simulink library "WECSim_Lib_update"  (Simulink 8.6)
settings: Solver=ode45  StartTime=0.0  StopTime=10.0  RelTol=1e-3
undefined symbols (not defined in the file or in its folder): body, constraint, mooring, pto, simu, waves, X, Y, Z
libraries: nesl_utility x168, sm_lib x94, vrlib x1
(part 5 of 6)

== system WECSim_Lib_update/Body Elements/Rigid Body/Hydrodynamic Body/Structure/Motion Sensor ==
  note: Measures the position, velocity, and acceleration of the follower (F) frame relative to the base (B) frame.
      | Ouputs a bus of 3 signals, each signal is a vector length 6.
  Angle : MATLAB Function  TreatAsAtomicUnit=on
  Bus Creator : BusCreator  Inputs=3
  Mux : Mux
  Mux1 : Mux  Inputs=6
  Mux2 : Mux  Inputs=6
  PS-Simulink Converter{,1..15} (16 alike) : nesl_utility/PS-Simulink Converter  PhysicalDomain=network_engine_domain  SubClassName=ps_output  LeftPortType=input  RightPortType=output  PseudoPeriodic=off  Frequencies=[]  AffineConversion=off
  Transform  Sensor : sm_lib/Frames and Transforms/Transform Sensor  MeasurementFrame=World  SenseAngle=off  SenseAxis=off  SenseAngle1=off  SenseAngle2=off  SenseAngle3=off  SenseQ=on  SenseR=off  SenseOmegaX=on  SenseOmegaY=on  SenseOmegaZ=on  SenseOmega1=off  SenseOmega2=off  SenseOmega3=off  SenseQDot=off  SenseRDot=off  SenseAlphaX=on  SenseAlphaY=on  SenseAlphaZ=on  SenseAlpha1=off  SenseAlpha2=off  SenseAlpha3=off  SenseQDDot=off  SenseRDDot=off  SenseX=on  SenseY=on  SenseZ=on  SenseRad=off  SenseAzim=off  SenseDist=off  SenseInc=off  SenseXDot=on  SenseYDot=on  SenseZDot=on  SenseRadDot=off  SenseAzimDot=off  SenseDistDot=off  SenseIncDot=off  SenseXDDot=on  SenseYDDot=on  SenseZDDot=on  SenseRadDDot=off  SenseAzimDDot=off  SenseDistDDot=off  SenseIncDDot=off
  F : PMIOPort  Port=1  Side=Right
  B : PMIOPort  Port=2  Side=Left
  Response : Outport
  wires:
  Bus Creator/1 -> Response/1
  PS-Simulink Converter15/1 -> Mux2/3  "az"
  PS-Simulink Converter3/1 -> Mux1/6  "omegaz"
  PS-Simulink Converter11/1 -> Mux1/2  "vy"
  PS-Simulink Converter2/1 -> Mux1/5  "omegay"
  PS-Simulink Converter1/1 -> Mux1/4  "omegax"
  PS-Simulink Converter6/1 -> Mux2/6  "alphaz"
  PS-Simulink Converter5/1 -> Mux2/5  "alphay"
  PS-Simulink Converter9/1 -> Mux/3  "z"
  PS-Simulink Converter8/1 -> Mux/2  "y"
  PS-Simulink Converter7/1 -> Mux/1  "x"
  Angle/1(E) -> Mux/4
  Mux2/1 -> Bus Creator/3  "acc"
  Mux1/1 -> Bus Creator/2  "vel"
  Mux/1 -> Bus Creator/1  "disp"
  PS-Simulink Converter14/1 -> Mux2/2  "ay"
  PS-Simulink Converter13/1 -> Mux2/1  "ax"
  PS-Simulink Converter12/1 -> Mux1/3  "vz"
  PS-Simulink Converter10/1 -> Mux1/1  "vx"
  PS-Simulink Converter4/1 -> Mux2/4  "alphax"
  PS-Simulink Converter/1 -> Angle/1(Q)
  connections:
  PS-Simulink Converter3/LConn1 -- Transform  Sensor/RConn5
  PS-Simulink Converter2/LConn1 -- Transform  Sensor/RConn4
  PS-Simulink Converter1/LConn1 -- Transform  Sensor/RConn3
  PS-Simulink Converter6/LConn1 -- Transform  Sensor/RConn8
  PS-Simulink Converter5/LConn1 -- Transform  Sensor/RConn7
  PS-Simulink Converter4/LConn1 -- Transform  Sensor/RConn6
  PS-Simulink Converter7/LConn1 -- Transform  Sensor/RConn9
  PS-Simulink Converter8/LConn1 -- Transform  Sensor/RConn10
  PS-Simulink Converter9/LConn1 -- Transform  Sensor/RConn11
  PS-Simulink Converter10/LConn1 -- Transform  Sensor/RConn12
  PS-Simulink Converter11/LConn1 -- Transform  Sensor/RConn13
  PS-Simulink Converter12/LConn1 -- Transform  Sensor/RConn14
  PS-Simulink Converter13/LConn1 -- Transform  Sensor/RConn15
  PS-Simulink Converter14/LConn1 -- Transform  Sensor/RConn16
  PS-Simulink Converter15/LConn1 -- Transform  Sensor/RConn17
  Transform  Sensor/RConn2 -- PS-Simulink Converter/LConn1
  B/RConn1 -- Transform  Sensor/LConn1
  Transform  Sensor/RConn1 -- F/RConn1

== system WECSim_Lib_update/Body Elements/Rigid Body/Hydrodynamic Body/Wave Diffraction and Excitation Force Calculation/Linear Wave Excitation Force Variant Subsystem ==
  note: 1) Add Subsystem or Model blocks as valid variant choices.
      | 2) You cannot connect blocks at this level. At simulation, connectivity is automatically
      | determined, based on the active variant and port name matching.
  In1 : Inport
  Irregular Wave  Excitation Force : Subsystem  VariantControl=sv_irregularWaves
  No Wave Excitation Force : Subsystem  VariantControl=sv_noWave
  Regular Wave  Excitation Force : Subsystem  VariantControl=sv_regularWaves
  User Defined Wave  Excitation Force : Subsystem  VariantControl=sv_udfWaves
  Out1 : Outport

== system WECSim_Lib_update/Body Elements/Rigid Body/Hydrodynamic Body/Wave Diffraction and Excitation Force Calculation/No Ramp Function ==
  Action Port : ActionPort
  Constant : Constant
  R : Outport  InitialOutput=1
  wires:
  Constant/1 -> R/1

== system WECSim_Lib_update/Body Elements/Rigid Body/Hydrodynamic Body/Wave Diffraction and Excitation Force Calculation/Nonlinear FK Force Variant Subsystem ==
  note: 1) Add Subsystem or Model blocks as valid variant choices.
      | 2) You cannot connect blocks at this level. At simulation, connectivity is automatically
      | determined, based on the active variant and port name matching.
  In1 : Inport
  In2 : Inport  Port=2
  In3 : Inport  Port=3
  No Nonlinear FroudeKrylov Force : Subsystem  VariantControl=sv_linearHydro
  With Nonlinear FroudeKrylov Force : Subsystem  TreatAsAtomicUnit=on  SystemSampleTime=simu.dtNL  VariantControl=sv_nonlinearHydro
  Out1 : Outport

== system WECSim_Lib_update/Body Elements/Rigid Body/Hydrodynamic Body/Wave Diffraction and Excitation Force Calculation/Ramp Function ==
  Time : Inport
  Action Port : ActionPort
  Add : Sum
  Add1 : Sum
  Constant : Constant  Value=1/2
  Constant1 : Constant
  Constant2 : Constant  Value=3*pi/2
  Constant3 : Constant  Value=pi
  Divide : Product  Inputs=*/
  Product : Product
  Product1 : Product
  Ramp Time : Constant  Value=simu.rampTime
  Sine Wave Function : Sin  TimeSource=Use external signal  SampleTime=0
  R : Outport
  wires:
  Add/1 -> Product/1
  Sine Wave Function/1 -> Add/2
  Constant1/1 -> Add/1
  Constant/1 -> Product/2
  Product/1 -> R/1
  Time/1 -> Product1/1  "t"
  Ramp Time/1 -> Divide/2  "t_ramp"
  Constant2/1 -> Add1/2  "phase"
  Add1/1 -> Sine Wave Function/1
  Product1/1 -> Add1/1
  Constant3/1 -> Divide/1
  Divide/1 -> Product1/2  "frequency"

== system WECSim_Lib_update/Body Elements/Rigid Body/Hydrodynamic Body/Wave Radiation Forces Calculation/SS CI and Constant-Damping-CoeVariant Subsystem ==
  note: 1) Add Subsystem or Model blocks as valid variant choices.
      | 2) You cannot connect blocks at this level. At simulation, connectivity is automatically
      | determined, based on the active variant and port name matching.
  In1 : Inport
  In2 : Inport  Port=2
  Constant Coefficients : Subsystem  VariantControl=sv_constantCoeff
  Convolution Integral Calculation : Subsystem  VariantControl=sv_convolution
  "State-Space Calculation " : Subsystem  VariantControl=sv_stateSpace
  Out1 : Outport

== system WECSim_Lib_update/Body Elements/Rigid Body/Non-Hydro Body/Structure/Motion Sensor ==
  note: Measures the position, velocity, and acceleration of the follower (F) frame relative to the base (B) frame.
      | Ouputs a bus of 3 signals, each signal is a vector length 6.
  Angle : MATLAB Function  TreatAsAtomicUnit=on
  Bus Creator : BusCreator  Inputs=3
  Mux : Mux
  Mux1 : Mux  Inputs=6
  Mux2 : Mux  Inputs=6
  PS-Simulink Converter{,1..15} (16 alike) : nesl_utility/PS-Simulink Converter  PhysicalDomain=network_engine_domain  SubClassName=ps_output  LeftPortType=input  RightPortType=output  PseudoPeriodic=off  Frequencies=[]  AffineConversion=off
  Transform  Sensor : sm_lib/Frames and Transforms/Transform Sensor  MeasurementFrame=World  SenseAngle=off  SenseAxis=off  SenseAngle1=off  SenseAngle2=off  SenseAngle3=off  SenseQ=on  SenseR=off  SenseOmegaX=on  SenseOmegaY=on  SenseOmegaZ=on  SenseOmega1=off  SenseOmega2=off  SenseOmega3=off  SenseQDot=off  SenseRDot=off  SenseAlphaX=on  SenseAlphaY=on  SenseAlphaZ=on  SenseAlpha1=off  SenseAlpha2=off  SenseAlpha3=off  SenseQDDot=off  SenseRDDot=off  SenseX=on  SenseY=on  SenseZ=on  SenseRad=off  SenseAzim=off  SenseDist=off  SenseInc=off  SenseXDot=on  SenseYDot=on  SenseZDot=on  SenseRadDot=off  SenseAzimDot=off  SenseDistDot=off  SenseIncDot=off  SenseXDDot=on  SenseYDDot=on  SenseZDDot=on  SenseRadDDot=off  SenseAzimDDot=off  SenseDistDDot=off  SenseIncDDot=off
  F : PMIOPort  Port=1  Side=Right
  B : PMIOPort  Port=2  Side=Left
  Response : Outport
  wires:
  Bus Creator/1 -> Response/1
  PS-Simulink Converter15/1 -> Mux2/3  "az"
  PS-Simulink Converter3/1 -> Mux1/6  "omegaz"
  PS-Simulink Converter11/1 -> Mux1/2  "vy"
  PS-Simulink Converter2/1 -> Mux1/5  "omegay"
  PS-Simulink Converter1/1 -> Mux1/4  "omegax"
  PS-Simulink Converter6/1 -> Mux2/6  "alphaz"
  PS-Simulink Converter5/1 -> Mux2/5  "alphay"
  PS-Simulink Converter9/1 -> Mux/3  "z"
  PS-Simulink Converter8/1 -> Mux/2  "y"
  PS-Simulink Converter7/1 -> Mux/1  "x"
  Angle/1(E) -> Mux/4
  Mux2/1 -> Bus Creator/3  "acc"
  Mux1/1 -> Bus Creator/2  "vel"
  Mux/1 -> Bus Creator/1  "disp"
  PS-Simulink Converter14/1 -> Mux2/2  "ay"
  PS-Simulink Converter13/1 -> Mux2/1  "ax"
  PS-Simulink Converter12/1 -> Mux1/3  "vz"
  PS-Simulink Converter10/1 -> Mux1/1  "vx"
  PS-Simulink Converter4/1 -> Mux2/4  "alphax"
  PS-Simulink Converter/1 -> Angle/1(Q)
  connections:
  PS-Simulink Converter3/LConn1 -- Transform  Sensor/RConn5
  PS-Simulink Converter2/LConn1 -- Transform  Sensor/RConn4
  PS-Simulink Converter1/LConn1 -- Transform  Sensor/RConn3
  PS-Simulink Converter6/LConn1 -- Transform  Sensor/RConn8
  PS-Simulink Converter5/LConn1 -- Transform  Sensor/RConn7
  PS-Simulink Converter4/LConn1 -- Transform  Sensor/RConn6
  PS-Simulink Converter7/LConn1 -- Transform  Sensor/RConn9
  PS-Simulink Converter8/LConn1 -- Transform  Sensor/RConn10
  PS-Simulink Converter9/LConn1 -- Transform  Sensor/RConn11
  PS-Simulink Converter10/LConn1 -- Transform  Sensor/RConn12
  PS-Simulink Converter11/LConn1 -- Transform  Sensor/RConn13
  PS-Simulink Converter12/LConn1 -- Transform  Sensor/RConn14
  PS-Simulink Converter13/LConn1 -- Transform  Sensor/RConn15
  PS-Simulink Converter14/LConn1 -- Transform  Sensor/RConn16
  PS-Simulink Converter15/LConn1 -- Transform  Sensor/RConn17
  Transform  Sensor/RConn2 -- PS-Simulink Converter/LConn1
  B/RConn1 -- Transform  Sensor/LConn1
  Transform  Sensor/RConn1 -- F/RConn1

== system WECSim_Lib_update/Moorings/MoorDyn/MoorDyn/MoorDyn/Triggered Subsystem ==
  X : Inport
  XD : Inport  Port=2
  Time : Inport  Port=3
  CoupTime : Inport  Port=4
  Trigger : TriggerPort  TriggerType=either
  MATLAB Function : MATLAB Function  TreatAsAtomicUnit=on
  FLines : Outport  PortDimensions=6
  wires:
  CoupTime/1 -> MATLAB Function/4(CoupTime)
  Time/1 -> MATLAB Function/3(Time)
  XD/1 -> MATLAB Function/2(XD)
  MATLAB Function/1(FLines) -> FLines/1
  X/1 -> MATLAB Function/1(X)

== system WECSim_Lib_update/Body Elements/Rigid Body/Hydrodynamic Body/B2B Subsystem/B2B/CrossCoupling ==
  note: CrossCoupling block is updated by its mask initialization, which is only called on when a simulation is run. 'From' blocks are automatically created and connected based on the number of bodies in the simulation.
  Mux1 : Mux  Inputs=2
  Mux2 : Mux  Inputs=2
  vel : Outport
  acc : Outport  Port=2
  wires:
  [vel1] -> Mux1/1
  Mux1/1 -> vel/1
  [vel2] -> Mux1/2
  [acc1] -> Mux2/1
  Mux2/1 -> acc/1
  [acc2] -> Mux2/2

== system WECSim_Lib_update/Body Elements/Rigid Body/Hydrodynamic Body/Hydrostatic Restoring Force Calculation/Linear and Nonlinear Restoring Force Variant Subsystem/Linear Hydrostatic Restoring Force  ==
  In1 : Inport
  Add1 : Sum  Inputs=+-
  Add2 : Sum  Inputs=+++
  Add3 : Sum  Inputs=+-
  Assignment (Add Net Bouyancy Force  to Z-Direction) : Assignment  IndexOptions=Index vector (dialog)  Indices=3  OutputSizes=1
  Assignment (Add Net Bouyancy Force  to Z-Direction)1 : Assignment  IndexOptions=Index vector (dialog)  Indices=3  OutputSizes=1
  Assignment (Add Net Bouyancy Force  to Z-Direction)2 : Assignment  IndexOptions=Index vector (dialog)  Indices=4:6  OutputSizes=1
  Body Mass : Constant  Value=body.hydroForce.storage.mass
  Center of Buoyancy : Constant  Value=body.cb
  Center of Gravity : Constant  Value=body.cg
  Constant1 : Constant  Value=[0 0 0 0 0 0]
  Constant2 : Constant  Value=[0 0 0]
  Cross Product : vrlib/Utilities/Cross Product
  Gravity : Constant  Value=simu.g
  Linear Restioring Coefficient Matrix : Constant  Value=body.hydroForce.linearHydroRestCoef
  Product : Product
  Product1 : Product  Inputs=3
  Product2 : Product  Multiplication=Matrix(*)
  Volume : Constant  Value=body.dispVol
  Water Density : Constant  Value=simu.rho
  Out1 : Outport
  wires:
  In1/1 -> Product2/2  "x"
  Body Mass/1 -> Product/2  "m"
  Assignment (Add Net Bouyancy Force  to Z-Direction)/1 -> Add2/1  "Net Buoyancy Force"
  Add2/1 -> Out1/1  "F_Restoring"
  Volume/1 -> Product1/3  "Vol"
  Gravity/1 -> Product1/2, Product/1  "g"
  Water Density/1 -> Product1/1  "rho"
  Product/1 -> Add1/1  "F_Gravity"
  Product1/1 -> Add1/2, Assignment (Add Net Bouyancy Force  to Z-Direction)1/2  "F_Buoyancy"
  Add1/1 -> Assignment (Add Net Bouyancy Force  to Z-Direction)/2
  Product2/1 -> Add2/2  "Linear Restoring Force"
  Linear Restioring Coefficient Matrix/1 -> Product2/1  "K"
  Center of Buoyancy/1 -> Add3/1  "x"
  Center of Gravity/1 -> Add3/2  "cg"
  Add3/1 -> Cross Product/2
  Constant2/1 -> Assignment (Add Net Bouyancy Force  to Z-Direction)1/1
  Assignment (Add Net Bouyancy Force  to Z-Direction)1/1 -> Cross Product/1
  Cross Product/1 -> Assignment (Add Net Bouyancy Force  to Z-Direction)2/2
  Constant1/1 -> Assignment (Add Net Bouyancy Force  to Z-Direction)2/1, Assignment (Add Net Bouyancy Force  to Z-Direction)/1
  Assignment (Add Net Bouyancy Force  to Z-Direction)2/1 -> Add2/3

== system WECSim_Lib_update/Body Elements/Rigid Body/Hydrodynamic Body/Hydrostatic Restoring Force Calculation/Linear and Nonlinear Restoring Force Variant Subsystem/Nonlinear Hydrostatic Restoring Force ==
  In1 : Inport
  In2 : Inport  Port=2
  Body Mass2 : Constant  Value=body.hydroForce.storage.mass
  Center of Gravity : Constant  Value=body.cg
  Gravity2 : Constant  Value=simu.g
  Rate Transition : RateTransition
  Rate Transition1 : RateTransition
  Restoring Forces : MATLAB Function  TreatAsAtomicUnit=on  SystemSampleTime=simu.dtNL
  STL areas : Constant  Value=body.bodyGeometry.area
  STL centers : Constant  Value=body.bodyGeometry.center
  STL normal vectors : Constant  Value=body.bodyGeometry.norm
  To Workspace1 : ToWorkspace  VariableName=body1_hspressure_out  SaveFormat=Structure With Time  SampleTime=-1
      settings: Decimation=round(simu.dtOut/simu.dt,0)
  Water Density1 : Constant  Value=simu.rho
  Out1 : Outport
  wires:
  In1/1 -> Restoring Forces/1(x)
  Center of Gravity/1 -> Restoring Forces/8(cg)
  Gravity2/1 -> Restoring Forces/7(g)  "g"
  Water Density1/1 -> Restoring Forces/6(rho)
  STL normal vectors/1 -> Restoring Forces/4(tnorm)
  STL centers/1 -> Restoring Forces/3(center)
  In2/1 -> Restoring Forces/2(elv)
  STL areas/1 -> Restoring Forces/5(area)
  Body Mass2/1 -> Restoring Forces/9(mass)
  Restoring Forces/2(p) -> Rate Transition1/1
  Rate Transition1/1 -> To Workspace1/1
  Restoring Forces/1(f) -> Rate Transition/1
  Rate Transition/1 -> Out1/1

== system WECSim_Lib_update/Body Elements/Rigid Body/Hydrodynamic Body/Morrison Element and ViscousDampingForceCalculation/Morrison Element Variant Subsystem/Morrison Element Off ==
  Constant : Constant  Value=[0 0 0 0 0 0]
  morison_force : Outport
  wires:
  Constant/1 -> morison_force/1

== system WECSim_Lib_update/Body Elements/Rigid Body/Hydrodynamic Body/Morrison Element and ViscousDampingForceCalculation/Morrison Element Variant Subsystem/Morrison Element On ==
  note: 1) Add Subsystem or Model blocks as valid variant choices.
      | 2) You cannot connect blocks at this level. At simulation, connectivity is automatically
      | determined, based on the active variant and port name matching.
  displacement : Inport
  velocity : Inport  Port=2
  acceleration : Inport  Port=3
  time : Inport  Port=4
  Irregular Wave  Morison Force : Subsystem  TreatAsAtomicUnit=on  SystemSampleTime=simu.dtME  VariantControl=sv_irregularWaves
  No Wave Morison Force : Subsystem  VariantControl=sv_noWave
  Regular Wave  Morison Force : Subsystem  TreatAsAtomicUnit=on  SystemSampleTime=simu.dtME  VariantControl=sv_regularWaves
  morison_force : Outport

== system WECSim_Lib_update/Body Elements/Rigid Body/Hydrodynamic Body/Nonlinear Wave Elevation/Linear or Instantaneous Free Surface/Instantaneous Water Free Surface   ==
  In1 : Inport
  In2 : Inport  Port=2
  Center of Gravity : Constant  Value=body.cg
  Frequency Spacing : Constant  Value=waves.dw
  Instantaneous FS : MATLAB Function  TreatAsAtomicUnit=on
  Ramp Time : Constant  Value=simu.rampTime
  STL Centers : Constant  Value=body.bodyGeometry.center
  Wave Amplitude : Constant  Value=waves.A
  Wave Direction : Constant  Value=waves.waveDir
  Wave Frequency : Constant  Value=waves.w
  Wave Number : Constant  Value=waves.k
  Wave Random Phase : Constant  Value=waves.phase
  Wave Type Number : Constant  Value=waves.typeNum
  Out1 : Outport
  wires:
  Instantaneous FS/1(f) -> Out1/1
  STL Centers/1 -> Instantaneous FS/2(center)
  Center of Gravity/1 -> Instantaneous FS/3(cg)
  Wave Number/1 -> Instantaneous FS/7(k)
  Wave Frequency/1 -> Instantaneous FS/5(w)
  Wave Type Number/1 -> Instantaneous FS/8(typeNum)
  Ramp Time/1 -> Instantaneous FS/10(rampT)
  Wave Random Phase/1 -> Instantaneous FS/11(phaseRand)
  Frequency Spacing/1 -> Instantaneous FS/6(dw)
  In2/1 -> Instantaneous FS/9(t)
  In1/1 -> Instantaneous FS/1(x)
  Wave Direction/1 -> Instantaneous FS/12(waveDir)
  Wave Amplitude/1 -> Instantaneous FS/4(AH)

== system WECSim_Lib_update/Body Elements/Rigid Body/Hydrodynamic Body/Nonlinear Wave Elevation/Linear or Instantaneous Free Surface/Mean Water Free Surface  ==
  zero : Constant  Value=0
  Out1 : Outport
  wires:
  zero/1 -> Out1/1

== system WECSim_Lib_update/Body Elements/Rigid Body/Hydrodynamic Body/Wave Diffraction and Excitation Force Calculation/Linear Wave Excitation Force Variant Subsystem/Irregular Wave  Excitation Force ==
  note: Calculates the wave force, F_wave, for the case of Irregular Waves.
      |
      | F_wave = sum( F_wave(i))
      |
      | where i = each frequency bin.
  In1 : Inport
  Frequency Spacing Delta Omega : Constant  Value=waves.dw  VectorParams1D=off
  Imaginary Part of Wave Excitation : Constant  Value=body.hydroForce.fExt.im  VectorParams1D=off
  MATLAB Function : MATLAB Function  TreatAsAtomicUnit=on
  Random Phase : Constant  Value=waves.phase  VectorParams1D=off
  Real Part of Wave Excitation : Constant  Value=body.hydroForce.fExt.re  VectorParams1D=off
  Wave Frequency : Constant  Value=waves.w  VectorParams1D=off
  Wave Spectrum : Constant  Value=waves.A  VectorParams1D=off
  Out1 : Outport
  wires:
  Random Phase/1 -> MATLAB Function/5(phaseRand)
  MATLAB Function/1(Fext) -> Out1/1
  Wave Frequency/1 -> MATLAB Function/2(w)
  Imaginary Part of Wave Excitation/1 -> MATLAB Function/4(fExtIM)
  Real Part of Wave Excitation/1 -> MATLAB Function/3(fExtRE)
  Wave Spectrum/1 -> MATLAB Function/1(A)
  In1/1 -> MATLAB Function/7(time)
  Frequency Spacing Delta Omega/1 -> MATLAB Function/6(dw)

== system WECSim_Lib_update/Body Elements/Rigid Body/Hydrodynamic Body/Wave Diffraction and Excitation Force Calculation/Linear Wave Excitation Force Variant Subsystem/No Wave Excitation Force ==
  Constant : Constant  Value=[0 0 0 0 0 0]
  Out1 : Outport
  wires:
  Constant/1 -> Out1/1

== system WECSim_Lib_update/Body Elements/Rigid Body/Hydrodynamic Body/Wave Diffraction and Excitation Force Calculation/Linear Wave Excitation Force Variant Subsystem/Regular Wave  Excitation Force ==
  note: Calculates the wave force, F_wave, for the case of Regular Waves.
      |
      | F_wave =   A * cos(w * t) * Re{Fext}
      |                -  A * sin(w * t) * Im{Fext}
  In1 : Inport
  Add : Sum
  Add1 : Sum  Inputs=+-
  Constant : Constant  Value=pi/2
  Excitation Imaginary Part : Constant  Value=body.hydroForce.fExt.im(1,:)  VectorParams1D=off
  Excitation Real Part : Constant  Value=body.hydroForce.fExt.re(1,:)  VectorParams1D=off
  Product : Product
  Product1 : Product  Inputs=3
  Product2 : Product  Inputs=3
  Sine Wave Function : Sin  TimeSource=Use external signal  SampleTime=0
  Sine Wave Function1 : Sin  TimeSource=Use external signal  SampleTime=0
  Wave Amplitude : Constant  Value=waves.A(1,:)
  Wave Frequency : Constant  Value=waves.w(1,:)
  Out1 : Outport
  wires:
  In1/1 -> Product/1  "t"
  Wave Frequency/1 -> Product/2  "w"
  Product/1 -> Sine Wave Function/1, Add/1
  Sine Wave Function1/1 -> Product1/3  "cos(w*t)"
  Sine Wave Function/1 -> Product2/2  "sin(wt)"
  Excitation Imaginary Part/1 -> Product2/3  "Im{Fext}"
  Excitation Real Part/1 -> Product1/2  "Re{Fext}"
  Product1/1 -> Add1/1
  Product2/1 -> Add1/2
  Add1/1 -> Out1/1
  Wave Amplitude/1 -> Product2/1, Product1/1  "A"
  Add/1 -> Sine Wave Function1/1
  Constant/1 -> Add/2

== system WECSim_Lib_update/Body Elements/Rigid Body/Hydrodynamic Body/Wave Diffraction and Excitation Force Calculation/Linear Wave Excitation Force Variant Subsystem/User Defined Wave  Excitation Force ==
  note: Calculates the wave force, F_wave, for the case of User Defined Waves.
      |
      | F_wave = convolution calculation [1x6]
  InputWaveForceTimeHistory : FromWorkspace  VariableName=[waves.waveAmpTime(:,1),body.hydroForce.userDefinedFe]  SampleTime=0
  Out1 : Outport
  wires:
  InputWaveForceTimeHistory/1 -> Out1/1

== system WECSim_Lib_update/Body Elements/Rigid Body/Hydrodynamic Body/Wave Diffraction and Excitation Force Calculation/Nonlinear FK Force Variant Subsystem/No Nonlinear FroudeKrylov Force ==
  Constant : Constant  Value=[0 0 0 0 0 0]
  Out1 : Outport
  wires:
  Constant/1 -> Out1/1

== system WECSim_Lib_update/Body Elements/Rigid Body/Hydrodynamic Body/Wave Diffraction and Excitation Force Calculation/Nonlinear FK Force Variant Subsystem/With Nonlinear FroudeKrylov Force ==
  In1 : Inport
  In2 : Inport  Port=2
  In3 : Inport  Port=3
  Add : Sum  Inputs=+-
  Center of Gravity : Constant  Value=body.hydroData.properties.cg
  Center of Gravity1 : Constant  Value=body.hydroData.properties.cg
  Constant : Constant  Value=[0 0 0]
  Deep Water Flag : Constant  Value=waves.deepWaterWave
  Diffraction and Excitation Forces : MATLAB Function  TreatAsAtomicUnit=on
  Frequency Spacing : Constant  Value=waves.dw
  Gravity : Constant  Value=simu.g
  Mux : Mux  Inputs=2
  STL Areas : Constant  Value=body.bodyGeometry.area
  STL Centers : Constant  Value=body.bodyGeometry.center
  STL Normal Vectors : Constant  Value=body.bodyGeometry.norm
  To Workspace : ToWorkspace  VariableName=body1_wavenonlinearpressure_out  SaveFormat=Structure With Time  SampleTime=-1
      settings: Decimation=round(simu.dtOut/simu.dt,0)
  To Workspace1 : ToWorkspace  VariableName=body1_wavelinearpressure_out  SaveFormat=Structure With Time  SampleTime=-1
      settings: Decimation=round(simu.dtOut/simu.dt,0)
  Water Density : Constant  Value=simu.rho
  Water Depth : Constant  Value=waves.waterDepth
  Wave Amplitude : Constant  Value=waves.A
  Wave Frequency : Constant  Value=waves.w
  Wave Number : Constant  Value=waves.k
  Wave Random Phase : Constant  Value=waves.phase
  Wave Type Number : Constant  Value=waves.typeNum
  Out1 : Outport
  wires:
  Center of Gravity1/1 -> Diffraction and Excitation Forces/8(cg)
  Diffraction and Excitation Forces/1(f) -> Out1/1
  Gravity/1 -> Diffraction and Excitation Forces/7(g)
  Water Density/1 -> Diffraction and Excitation Forces/6(rho)
  STL Normal Vectors/1 -> Diffraction and Excitation Forces/4(tnorm)
  STL Centers/1 -> Diffraction and Excitation Forces/3(center)
  In3/1 -> Diffraction and Excitation Forces/2(elv)
  In1/1 -> Diffraction and Excitation Forces/16(t)
  Wave Amplitude/1 -> Diffraction and Excitation Forces/9(AH)
  Wave Frequency/1 -> Diffraction and Excitation Forces/10(w)
  Frequency Spacing/1 -> Diffraction and Excitation Forces/11(dw)
  Wave Type Number/1 -> Diffraction and Excitation Forces/15(typeNum)
  Wave Number/1 -> Diffraction and Excitation Forces/14(k)
  Water Depth/1 -> Diffraction and Excitation Forces/12(wDepth)
  Wave Random Phase/1 -> Diffraction and Excitation Forces/17(phaseRand)
  Deep Water Flag/1 -> Diffraction and Excitation Forces/13(deepWaterWave)
  Add/1 -> Diffraction and Excitation Forces/1(x)  "x_cg"
  Mux/1 -> Add/2
  Center of Gravity/1 -> Mux/1  "cg"
  Constant/1 -> Mux/2
  In2/1 -> Add/1
  Diffraction and Excitation Forces/3(wpMeanFS) -> To Workspace1/1
  Diffraction and Excitation Forces/2(wp) -> To Workspace/1
  STL Areas/1 -> Diffraction and Excitation Forces/5(area)

== system WECSim_Lib_update/Body Elements/Rigid Body/Hydrodynamic Body/Wave Radiation Forces Calculation/SS CI and Constant-Damping-CoeVariant Subsystem/Constant Coefficients ==
  In1 : Inport
  Product : Product  Multiplication=Matrix(*)
  Radiation Damping Matrix : Constant  Value=body.hydroForce.fDamping
  Out1 : Outport
  wires:
  Radiation Damping Matrix/1 -> Product/1
  Product/1 -> Out1/1  "F_Single Frequency"
  In1/1 -> Product/2

== system WECSim_Lib_update/Body Elements/Rigid Body/Hydrodynamic Body/Wave Radiation Forces Calculation/SS CI and Constant-Damping-CoeVariant Subsystem/Convolution Integral Calculation ==
  In1 : Inport
  MATLAB Function : MATLAB Function  TreatAsAtomicUnit=on  SystemSampleTime=simu.CTTime(2) - simu.CTTime(1)  mask{IRKB=body.hydroForce.irkb, lenJ=length(body.lenJ), CTTime=simu.CTTime}
  Rate Transition : RateTransition
  Reshape : Reshape
  Out1 : Outport
  wires:
  In1/1 -> MATLAB Function/1(v)
  Reshape/1 -> Out1/1
  MATLAB Function/1(F_FM) -> Rate Transition/1
  Rate Transition/1 -> Reshape/1

== system WECSim_Lib_update/Body Elements/Rigid Body/Hydrodynamic Body/Wave Radiation Forces Calculation/SS CI and Constant-Damping-CoeVariant Subsystem/State-Space Calculation  ==
  In1 : Inport
  State-Space : StateSpace  A=body.hydroForce.ssRadf.A  B=body.hydroForce.ssRadf.B  C=body.hydroForce.ssRadf.C  D=body.hydroForce.ssRadf.D  X0=0
  Out1 : Outport
  wires:
  In1/1 -> State-Space/1  "x"
  State-Space/1 -> Out1/1

== system WECSim_Lib_update/Body Elements/Rigid Body/Hydrodynamic Body/Morrison Element and ViscousDampingForceCalculation/Morrison Element Variant Subsystem/Morrison Element On/Irregular Wave  Morison Force ==
  displacement : Inport
  velocity : Inport  Port=2
  acceleration : Inport  Port=3
  time : Inport  Port=4
  Area : Constant  Value=body.morrisonElement.characteristicArea  VectorParams1D=off
  Ca : Constant  Value=body.morrisonElement.ca  VectorParams1D=off
  Cd : Constant  Value=body.morrisonElement.cd  VectorParams1D=off
  Density : Constant  Value=simu.rho
  Gravity : Constant  Value=simu.g
  "MorrisonElement(s) " : MATLAB Function  TreatAsAtomicUnit=on
  Ramp Function Time : Constant  Value=simu.rampTime
  RandomPhaseAngle : Constant  Value=waves.phase  VectorParams1D=off
  Volume : Constant  Value=body.morrisonElement.VME  VectorParams1D=off
  WaterDepth : Constant  Value=waves.waterDepth
  WaveAmp : Constant  Value=waves.A
  WaveFreq : Constant  Value=waves.w
  WaveHeading : Constant  Value=waves.waveDir
  WaveNumber : Constant  Value=waves.k
  dw : Constant  Value=waves.dw  VectorParams1D=off
  "r_{g}" : Constant  Value=body.morrisonElement.rgME  VectorParams1D=off
  morison_force : Outport
  wires:
  Volume/1 -> "MorrisonElement(s) "/7(Vol)
  acceleration/1 -> "MorrisonElement(s) "/3(Accel)
  displacement/1 -> "MorrisonElement(s) "/4(Disp)
  Area/1 -> "MorrisonElement(s) "/5(Area)
  "r_{g}"/1 -> "MorrisonElement(s) "/1(r)
  velocity/1 -> "MorrisonElement(s) "/2(Vel)
  WaterDepth/1 -> "MorrisonElement(s) "/12(waterDepth)
  Gravity/1 -> "MorrisonElement(s) "/17(g)
  WaveNumber/1 -> "MorrisonElement(s) "/13(k)
  WaveHeading/1 -> "MorrisonElement(s) "/11(waveDir)
  time/1 -> "MorrisonElement(s) "/9(Time)
  Density/1 -> "MorrisonElement(s) "/10(rho)
  RandomPhaseAngle/1 -> "MorrisonElement(s) "/18(randPhase)
  WaveFreq/1 -> "MorrisonElement(s) "/14(w)
  Ca/1 -> "MorrisonElement(s) "/8(Ca)
  dw/1 -> "MorrisonElement(s) "/19(dw)
  WaveAmp/1 -> "MorrisonElement(s) "/15(A)
  Cd/1 -> "MorrisonElement(s) "/6(Cd)
  Ramp Function Time/1 -> "MorrisonElement(s) "/16(rampTime)
  "MorrisonElement(s) "/1(f) -> morison_force/1

== system WECSim_Lib_update/Body Elements/Rigid Body/Hydrodynamic Body/Morrison Element and ViscousDampingForceCalculation/Morrison Element Variant Subsystem/Morrison Element On/No Wave Morison Force ==
  displacement : Inport
  velocity : Inport  Port=2
  acceleration : Inport  Port=3
  time : Inport  Port=4
  Area : Constant  Value=body.morrisonElement.characteristicArea  VectorParams1D=off
  Ca : Constant  Value=body.morrisonElement.ca  VectorParams1D=off
  Cd : Constant  Value=body.morrisonElement.cd  VectorParams1D=off
  Density : Constant  Value=simu.rho
  "MorrisonElement(s) " : MATLAB Function  TreatAsAtomicUnit=on
  Terminator : Terminator
  Volume : Constant  Value=body.morrisonElement.VME  VectorParams1D=off
  "r_{g}" : Constant  Value=body.morrisonElement.rgME  VectorParams1D=off
  morison_force : Outport
  wires:
  "MorrisonElement(s) "/1(f) -> morison_force/1
  acceleration/1 -> "MorrisonElement(s) "/3(Accel)
  Density/1 -> "MorrisonElement(s) "/9(rho)
  Volume/1 -> "MorrisonElement(s) "/7(Vol)
  "r_{g}"/1 -> "MorrisonElement(s) "/1(r)
  Ca/1 -> "MorrisonElement(s) "/8(Ca)
  Area/1 -> "MorrisonElement(s) "/5(Area)
  displacement/1 -> "MorrisonElement(s) "/4(Disp)
  Cd/1 -> "MorrisonElement(s) "/6(Cd)
  velocity/1 -> "MorrisonElement(s) "/2(Vel)
  time/1 -> Terminator/1

== system WECSim_Lib_update/Body Elements/Rigid Body/Hydrodynamic Body/Morrison Element and ViscousDampingForceCalculation/Morrison Element Variant Subsystem/Morrison Element On/Regular Wave  Morison Force ==
  displacement : Inport
  velocity : Inport  Port=2
  acceleration : Inport  Port=3
  time : Inport  Port=4
  Area : Constant  Value=body.morrisonElement.characteristicArea  VectorParams1D=off
  Ca : Constant  Value=body.morrisonElement.ca  VectorParams1D=off
  Cd : Constant  Value=body.morrisonElement.cd  VectorParams1D=off
  Density : Constant  Value=simu.rho
  Gravity : Constant  Value=simu.g
  "MorrisonElement(s) " : MATLAB Function  TreatAsAtomicUnit=on
  Ramp Function Time : Constant  Value=simu.rampTime
  Volume : Constant  Value=body.morrisonElement.VME  VectorParams1D=off
  WaterDepth : Constant  Value=waves.waterDepth
  WaveAmp : Constant  Value=waves.A
  WaveFreq : Constant  Value=waves.w
  WaveHeading : Constant  Value=waves.waveDir
  WaveNumber : Constant  Value=waves.k
  "r_{g}" : Constant  Value=body.morrisonElement.rgME  VectorParams1D=off
  morison_force : Outport
  wires:
  "MorrisonElement(s) "/1(f) -> morison_force/1
  Volume/1 -> "MorrisonElement(s) "/7(Vol)
  Ca/1 -> "MorrisonElement(s) "/8(Ca)
  Gravity/1 -> "MorrisonElement(s) "/17(g)
  Cd/1 -> "MorrisonElement(s) "/6(Cd)
  displacement/1 -> "MorrisonElement(s) "/4(Disp)
  WaveAmp/1 -> "MorrisonElement(s) "/15(A)
  WaveFreq/1 -> "MorrisonElement(s) "/14(w)
  Density/1 -> "MorrisonElement(s) "/10(rho)
  acceleration/1 -> "MorrisonElement(s) "/3(Accel)
  velocity/1 -> "MorrisonElement(s) "/2(Vel)
  WaveHeading/1 -> "MorrisonElement(s) "/11(waveDir)
  WaveNumber/1 -> "MorrisonElement(s) "/13(k)
  Ramp Function Time/1 -> "MorrisonElement(s) "/16(rampTime)
  time/1 -> "MorrisonElement(s) "/9(Time)
  WaterDepth/1 -> "MorrisonElement(s) "/12(waterDepth)
  "r_{g}"/1 -> "MorrisonElement(s) "/1(r)
  Area/1 -> "MorrisonElement(s) "/5(Area)

== matlab function Body Elements/Rigid Body/Hydrodynamic Body/Hydrostatic Restoring Force Calculation/Linear and Nonlinear Restoring Force Variant Subsystem/Nonlinear Hydrostatic Restoring Force/Restoring Forces ==
  data: x input double; elv input double; center input double; f output double; tnorm input double; area input double; rho input double; g input double; cg input double; p output double; mass input double
function [f,p]  = nonLinearBuoyancy(x,elv,center,tnorm,area,rho,g,cg,mass)
% Function to calculate buoyancy force and moment on a triangulated surface
% NOTE: This function assumes that the STL file is imported with its CG at 0,0,0
[f,p] = calc_buoyancy(x,elv,center,tnorm,area,rho,g,cg);
f = -f + [0 0 g*mass 0 0 0]';
end


function [f,p] = calc_buoyancy(x,elv,center,tnorm,area,rho,g,cg)
% Function to apply translation and rotation and calculate forces

% Compute new tri coords after cog rotation and translation
center = rotateXYZ(center,[1 0 0],x(4));
center = rotateXYZ(center,[0 1 0],x(5));
center = rotateXYZ(center,[0 0 1],x(6));
center = offsetXYZ(center,x);
center = offsetXYZ(center,cg);
% Compute new normal vectors coords after cog rotation
tnorm = rotateXYZ(tnorm,[1 0 0],x(4));
tnorm = rotateXYZ(tnorm,[0 1 0],x(5));
tnorm = rotateXYZ(tnorm,[0 0 1],x(6));

% Calculate the hydrostatic forces
av = tnorm .* [area area area];
[f,p]=fHydrostatic(center,elv,x(1:3)+cg,av,rho,g);
end

function verts = offsetXYZ(verts,x)
% Function to move the position vertices
verts(:,1) = verts(:,1) + x(1);
verts(:,2) = verts(:,2) + x(2);
verts(:,3) = verts(:,3) + x(3);
end

function xn = rotateXYZ(x,ax,t)
% Function to rotate a point about an arbitrary axis
% x: 3-componenet coordiantes
% ax: axis about which to rotate (must be a vector length 1)
% t: rotation angle
% xn: new coordinates after rotation
rotMat = zeros(3);
rotMat(1,1) = ax(1)*ax(1)*(1-cos(t))    + cos(t);
rotMat(1,2) = ax(2)*ax(1)*(1-cos(t))    + ax(3)*sin(t);
rotMat(1,3) = ax(3)*ax(1)*(1-cos(t))    - ax(2)*sin(t);
rotMat(2,1) = ax(1)*ax(2)*(1-cos(t))    - ax(3)*sin(t);
rotMat(2,2) = ax(2)*ax(2)*(1-cos(t))    + cos(t);
rotMat(2,3) = ax(3)*ax(2)*(1-cos(t))    + ax(1)*sin(t);
rotMat(3,1) = ax(1)*ax(3)*(1-cos(t))    + ax(2)*sin(t);
rotMat(3,2) = ax(2)*ax(3)*(1-cos(t))    - ax(1)*sin(t);
rotMat(3,3) = ax(3)*ax(3)*(1-cos(t))    + cos(t);
xn = x*rotMat;
end

function [f,p] = fHydrostatic(center,elv,instcg,av,rho,g)
% Function to calculate the force and moment about the cog due to hydrostatic pressure
f = zeros(6,1);

% Zeor out regions above the mean free surface
z=center(:,3); z((z-elv)>0)=0;

% Calculate the hydrostatic pressure at each triangle center
pressureVect = rho*g.*[-z -z -z].*-av;
p = rho*g.*-z;
% Compute force about cog
f(1:3) = sum(pressureVect);

tmp1 = ones(length(center(:,1)),1);
tmp2 = tmp1*instcg';
center2cgVec = center-tmp2;

f(4:6)= sum(cross(center2cgVec,pressureVect));
end

== matlab function Body Elements/Rigid Body/Hydrodynamic Body/Wave Radiation Forces Calculation/SS CI and Constant-Damping-CoeVariant Subsystem/Convolution Integral Calculation/MATLAB Function ==
  data: v input double; F_FM output double size=[6 1]; IRKB parameter double; lenJ parameter double size=1; CTTime parameter double
function F_FM = ConvolutionIntegral_interp(v, IRKB, lenJ, CTTime)
%#codegen
% Function to calculate convolution integral

%define persistent variables
interp_factor = 1;
persistent velocity IRKB_interp CTTime_interp;

if isempty(velocity) 
    CTTime_interp  = CTTime(1:interp_factor:end);
    velocity       = zeros(lenJ,length(CTTime_interp));
    IRKB_reordered = permute(IRKB,[3 1 2]);                     % permutes from [601 6 12] to [12 601 6]
    IRKB_interp    = IRKB_reordered(:,1:interp_factor:end, :);  % what does this do?
end 
% shift velocity
velocity      = circshift(velocity, 1, 2);
v = v(:)'';           %force v to be a column
velocity(:,1) = v(:);

%integrate
time_series = bsxfun(@times, IRKB_interp, velocity);
F_FM = squeeze(trapz(CTTime_interp,sum(time_series, 1)));

end

== matlab function Body Elements/Rigid Body/Hydrodynamic Body/Morrison Element and ViscousDampingForceCalculation/Morrison Element Variant Subsystem/Morrison Element On/No Wave Morison Force/MorrisonElement(s)  ==
  data: r input double; f output double; Vel input double; Accel input double; Disp input double; Area input double; Cd input double; Vol input double; Ca input double; rho input double
function f = fcn(r,Vel,Accel,Disp,Area,Cd,Vol,Ca,rho)
[rr,~]=size(r);
FMt = zeros(rr,6);
for ii = 1:rr
% Calculate Rotation Matrix
RotMax = [cos(Disp(5))*cos(Disp(6)) , cos(Disp(4))*sin(Disp(6)) + sin(Disp(4))*sin(Disp(5))*cos(Disp(6)) , sin(Disp(4))*sin(Disp(6)) - cos(Disp(4))*sin(Disp(5))*sin(Disp(6));...
          -cos(Disp(5))*sin(Disp(6)), cos(Disp(4))*cos(Disp(6)) -  sin(Disp(4))*sin(Disp(5))*sin(Disp(6)), sin(Disp(4))*cos(Disp(6)) + cos(Disp(4))*sin(Disp(5))*sin(Disp(6));...
          sin(Disp(5))              , -sin(Disp(4))*cos(Disp(5))                                         , cos(Disp(4))*cos(Disp(5))                                        ];
% Rotate Cartesian 
rRot    = mtimes(r(ii,:),RotMax);
Dispt   = [Disp(1),Disp(2),Disp(3)]; 
ShiftCg = Dispt + rRot;
% Update translational and rotational velocity
Velt    = [Vel(4),Vel(5),Vel(6)];                       % w refers to \omega = rotational velocity
wxr     = cross(Velt,r(ii,:)); 
%Vel should be a column vector
Vel2    = [Vel(1),Vel(2),Vel(3)] + wxr;
% Update translational and rotational acceleration
Accelt  = [Accel(4),Accel(5),Accel(6)];
dotwxr  = cross(Accelt,r(ii,:));                        % dotw refers to \dot{\omega} = rotational acceleration
wxwxr   = cross(Velt,wxr);
Accel2  = [Accel(1),Accel(2),Accel(3)] + dotwxr + wxwxr;
%% Added inertia and drag forces
areaRot = abs(mtimes(Area(ii,:),RotMax));
CdRot   = mtimes(abs(Cd(ii,:)),RotMax);
CaRot   = abs(mtimes(Ca(ii,:),RotMax));
% Forces from body velocity drag
FxuV    = (1/2)*abs(-1*Vel2(1))*-1*Vel2(1)*rho*CdRot(1)*areaRot(1);
FxvV    = (1/2)*abs(-1*Vel2(2))*-1*Vel2(2)*rho*CdRot(2)*areaRot(2);
FxwV    = (1/2)*abs(-1*Vel2(3))*-1*Vel2(3)*rho*CdRot(3)*areaRot(3);
% Forces from body acceleration inertia 
FxuA = rho*Vol(ii,:)*CaRot(1)*-1*Accel2(1); 
FxvA = rho*Vol(ii,:)*CaRot(2)*-1*Accel2(2);
FxwA = rho*Vol(ii,:)*CaRot(3)*-1*Accel2(3);
% Sum the force and moment contributions
if ShiftCg(3) > 0
    FMt(ii,:)   = [0, 0, 0, 0, 0, 0];
else
    F           = [FxuV + FxuA,...
                   FxvV + FxvA,...
                   FxwV + FxwA];
    M           = cross(rRot,F);
    FMt(ii,:)   = [F,M];
end
end
f  = [sum(FMt(:,1));sum(FMt(:,2));sum(FMt(:,3));sum(FMt(:,4));sum(FMt(:,5));sum(FMt(:,6))];

== matlab function Body Elements/Rigid Body/Hydrodynamic Body/Morrison Element and ViscousDampingForceCalculation/Morrison Element Variant Subsystem/Morrison Element On/Regular Wave Morison Force/MorrisonElement(s)  ==
  data: r input double; f output double; Vel input double; Accel input double; Disp input double; Area input double; Cd input double; Vol input double; Ca input double; Time input double; rho input double; waveDir input double; waterDepth input double; k input double; w input double; A input double; rampTime input double; g input double
function f = fcn(r,Vel,Accel,Disp,Area,Cd,Vol,Ca,Time,rho,waveDir,waterDepth,k,w,A,rampTime,g)
[rr,~]=size(r);
FMt = zeros(rr,6);
for ii = 1:rr
    % Calculate Rotation Matrix
    RotMax = [cos(Disp(5))*cos(Disp(6)) , cos(Disp(4))*sin(Disp(6)) + sin(Disp(4))*sin(Disp(5))*cos(Disp(6)) , sin(Disp(4))*sin(Disp(6)) - cos(Disp(4))*sin(Disp(5))*sin(Disp(6));...
        -cos(Disp(5))*sin(Disp(6)), cos(Disp(4))*cos(Disp(6)) -  sin(Disp(4))*sin(Disp(5))*sin(Disp(6)), sin(Disp(4))*cos(Disp(6)) + cos(Disp(4))*sin(Disp(5))*sin(Disp(6));...
        sin(Disp(5))              , -sin(Disp(4))*cos(Disp(5))                                         , cos(Disp(4))*cos(Disp(5))                                        ];
    % Rotate Cartesian
    rRot    = mtimes(r(ii,:),RotMax);
    Dispt   = [Disp(1),Disp(2),Disp(3)];
    ShiftCg = Dispt + rRot;
    % Update translational and rotational velocity
    % w refers to \omega = rotational velocity
    Velt    = [Vel(4),Vel(5),Vel(6)];
    wxr     = cross(Velt,r(ii,:));
    %Vel should be a column vector
    Vel2    = [Vel(1),Vel(2),Vel(3)] + wxr;
    % Update translational and rotational acceleration
    % dotw refers to \dot{\omega} = rotational acceleration
    Accelt  = [Accel(4),Accel(5),Accel(6)];
    dotwxr  = cross(Accelt,r(ii,:));
    wxwxr   = cross(Velt,wxr);
    Accel2  = [Accel(1),Accel(2),Accel(3)] + dotwxr + wxwxr;
    %% Calculate Orbital Velocity
    waveDirRad     = waveDir*pi/180;
    phaseArg       = w*Time - k*(ShiftCg(1)*cos(waveDirRad) + ShiftCg(2)*sin(waveDirRad));
    % Vertical Variation
    kh              = k*waterDepth;
    kz              = k*ShiftCg(3);
    if kh > pi  % Deep water wave
        coeffHorz  = exp(kz);
        coeffVert  = coeffHorz;
    else        % Shallow & Intermediate Depth
        coeffHorz  = cosh(kz + kh)/cosh(kh);
        coeffVert  = sinh(kz + kh)/cosh(kh);
    end
    % Ramp Time
    if Time <= rampTime
        ramp        = (A/2)*(1 + cos( pi + pi/rampTime*Time));
    else
        ramp        = A;
    end
    % Orbital Velocity
    uV              =  ramp*coeffHorz*cos(phaseArg)*g*k*(1/w)*cos(waveDirRad);
    vV              =  ramp*coeffHorz*cos(phaseArg)*g*k*(1/w)*sin(waveDirRad);
    wV              = -ramp*coeffVert*sin(phaseArg)*g*k*(1/w);
    % Orbital Acceleration
    uA              = -ramp*coeffHorz*sin(phaseArg)*g*k*cos(waveDirRad);
    vA              = -ramp*coeffHorz*sin(phaseArg)*g*k*sin(waveDirRad);
    wA              = -ramp*coeffVert*cos(phaseArg)*g*k;
    %% Added inertia and drag forces
    areaRot         = abs(mtimes(Area(ii,:),RotMax));
    CdRot           = mtimes(abs(Cd(ii,:)),RotMax);
    CaRot           = abs(mtimes(Ca(ii,:),RotMax));
    % Forces from velocity drag
    uVdiff          = uV - Vel2(1); FxuV = (1/2)*abs(uVdiff)*uVdiff*rho*CdRot(1)*areaRot(1);
    vVdiff          = vV - Vel2(2); FxvV = (1/2)*abs(vVdiff)*vVdiff*rho*CdRot(2)*areaRot(2);
    wVdiff          = wV - Vel2(3); FxwV = (1/2)*abs(wVdiff)*wVdiff*rho*CdRot(3)*areaRot(3);
    % Forces from body acceleration inertia
    uAdiff          = uA - Accel2(1); FxuA = uAdiff*rho*Vol(ii,:)*CaRot(1);
    vAdiff          = vA - Accel2(2); FxvA = vAdiff*rho*Vol(ii,:)*CaRot(2);
    wAdiff          = wA - Accel2(3); FxwA = wAdiff*rho*Vol(ii,:)*CaRot(3);
    % Forces from fluid acceleration inertia
    FxuAf           = uA*Vol(ii,:)*rho;
    FxvAf           = vA*Vol(ii,:)*rho;
    FxwAf           = wA*Vol(ii,:)*rho;
    % Sum the three force contributions
    if ShiftCg(3) > 0
        F           = [0, 0, 0];
        M           = [0, 0, 0];
        FMt(ii,:)   = [F,M];
    else
        F           = [FxuV + FxuA + FxuAf,...
            FxvV + FxvA + FxvAf,...
            FxwV + FxwA + FxwAf];
        M           = cross(rRot,F);
        FMt(ii,:)   = [F,M];
    end
end
f  = [sum(FMt(:,1));sum(FMt(:,2));sum(FMt(:,3));sum(FMt(:,4));sum(FMt(:,5));sum(FMt(:,6))];

== matlab function Moorings/MoorDyn/Structure/Motion Sensor/Angle ==
  data: Q input double; E output double
function E  = EulerAngle(Q)
%#codegen
E=zeros(3,1);
E(1) = atan2( (2*(Q(1)*Q(2)+Q(3)*Q(4))), (1-2* (Q(2)^2+Q(3)^2) ) );
E(2) = asin( 2* (Q(1)*Q(3) - Q(4)*Q(2)));
E(3) = atan2( (2*(Q(1)*Q(4)+Q(2)*Q(3))), (1-2* (Q(3)^2+Q(4)^2) ) );

== matlab function Moorings/MoorDyn/MoorDyn/MoorDyn/Triggered Subsystem/MATLAB Function ==
  data: X input double; FLines output double; XD input double; Time input double; CoupTime input double
function FLines  = MoorDyn_matlab_FCN(X,XD,Time,CoupTime)

    FLines = zeros(1,6);
    coder.extrinsic('MoorDyn_caller');
    
    FLines = MoorDyn_caller(X,XD,Time-CoupTime,CoupTime);

== matlab function Body Elements/Rigid Body/Hydrodynamic Body/Morrison Element and ViscousDampingForceCalculation/Morrison Element Variant Subsystem/Morrison Element On/Irregular Wave Morison Force/MorrisonElement(s)  ==
  data: r input double; f output double; Vel input double; Accel input double; Disp input double; Area input double; Cd input double; Vol input double; Ca input double; Time input double; rho input double; waveDir input double; waterDepth input double; k input double; w input double; A input double; rampTime input double; g input double; randPhase input double; dw input double
function f = fcn(r,Vel,Accel,Disp,Area,Cd,Vol,Ca,Time,rho,waveDir,waterDepth,k,w,A,rampTime,g,randPhase,dw)
[rr,~]  = size(r); [ff]    = length(w);
FMt     = zeros(rr,6);
uVt     = zeros(ff,1); vVt = uVt; wVt = vVt; uAt = wVt; vAt = uAt; wAt = vAt;
for ii = 1:rr
    % Calculate Rotation Matrix
    RotMax = [cos(Disp(5))*cos(Disp(6)) , cos(Disp(4))*sin(Disp(6)) + sin(Disp(4))*sin(Disp(5))*cos(Disp(6)) , sin(Disp(4))*sin(Disp(6)) - cos(Disp(4))*sin(Disp(5))*sin(Disp(6));...
              -cos(Disp(5))*sin(Disp(6)), cos(Disp(4))*cos(Disp(6)) -  sin(Disp(4))*sin(Disp(5))*sin(Disp(6)), sin(Disp(4))*cos(Disp(6)) + cos(Disp(4))*sin(Disp(5))*sin(Disp(6));...
              sin(Disp(5))              , -sin(Disp(4))*cos(Disp(5))                                         , cos(Disp(4))*cos(Disp(5))                                        ];
    % Rotate Cartesian
    rRot    = mtimes(r(ii,:),RotMax);
    Dispt   = [Disp(1),Disp(2),Disp(3)];
    ShiftCg = Dispt + rRot;
    % Update translational and rotational velocity
    % w refers to \omega = rotational velocity
    Velt    = [Vel(4),Vel(5),Vel(6)];
    wxr     = cross(Velt,r(ii,:));
    % Update Translational Velocity
    Vel2    = [Vel(1),Vel(2),Vel(3)] + wxr;
    % Update translational and rotational acceleration
    % dotw refers to \dot{\omega} = rotational acceleration
    Accelt  = [Accel(4),Accel(5),Accel(6)];
    dotwxr  = cross(Accelt,r(ii,:));
    wxwxr   = cross(Velt,wxr);
    % Update Translational Acceleration
    Accel2  = [Accel(1),Accel(2),Accel(3)] + dotwxr + wxwxr;
    %% Calculate Orbital Velocity
    for jj = 1:ff
        waveDirRad      = waveDir*pi/180;
        phaseArg        = w(jj,1)*Time - k(jj,1)*(ShiftCg(1)*cos(waveDirRad) + ShiftCg(2)*sin(waveDirRad)) + randPhase(jj,1);
        % Vertical Variation
        kh              = k(jj,1)*waterDepth;
        kz              = k(jj,1)*ShiftCg(3);
        if kh > pi % Deep Water Wave
            coeffHorz  = exp(kz);
            coeffVert  = coeffHorz;
        else % Shallow & Intermediate depth
            coeffHorz  = cosh(kz + kh)/cosh(kh);
            coeffVert  = sinh(kz + kh)/cosh(kh);
        end
        % Ramp Time
        if Time <= rampTime
            ramp        = (sqrt(A(jj,1)*dw(jj,1))/2)*(1 + cos(pi + pi/rampTime*Time));
        else
            ramp        = sqrt(A(jj,1)*dw(jj,1));
        end
        % Orbital Velocity for each individual wave component
        uVt(jj,1)       =  ramp*coeffHorz*cos(phaseArg)*g*k(jj,1)*(1/w(jj,1))*cos(waveDirRad);
        vVt(jj,1)       =  ramp*coeffHorz*cos(phaseArg)*g*k(jj,1)*(1/w(jj,1))*sin(waveDirRad);
        wVt(jj,1)       = -ramp*coeffVert*sin(phaseArg)*g*k(jj,1)*(1/w(jj,1));
        % Orbital Acceleration for each individual wave component
        uAt(jj,1)       = -ramp*coeffHorz*sin(phaseArg)*g*k(jj,1)*cos(waveDirRad);
        vAt(jj,1)       = -ramp*coeffHorz*sin(phaseArg)*g*k(jj,1)*sin(waveDirRad);
        wAt(jj,1)       = -ramp*coeffVert*cos(phaseArg)*g*k(jj,1);
    end
    % Sum the wave components to obtain the x, y, z orbital velocities
    uV = sum(uVt); uA = sum(uAt); vV = sum(vVt); vA = sum(vAt); wV = sum(wVt); wA = sum(wAt);
    %% Added inertia and drag forces
    areaRot         = abs(mtimes(Area(ii,:),RotMax));
    CdRot           = mtimes(abs(Cd(ii,:)),RotMax);
    CaRot           = abs(mtimes(Ca(ii,:),RotMax));
    % Forces from velocity drag
    uVdiff          = uV - Vel2(1); FxuV = (1/2)*abs(uVdiff)*uVdiff*rho*CdRot(1)*areaRot(1);
    vVdiff          = vV - Vel2(2); FxvV = (1/2)*abs(vVdiff)*vVdiff*rho*CdRot(2)*areaRot(2);
    wVdiff          = wV - Vel2(3); FxwV = (1/2)*abs(wVdiff)*wVdiff*rho*CdRot(3)*areaRot(3);
    % Forces from body acceleration inertia
    uAdiff          = uA - Accel2(1); FxuA = uAdiff*rho*Vol(ii,:)*CaRot(1);
    vAdiff          = vA - Accel2(2); FxvA = vAdiff*rho*Vol(ii,:)*CaRot(2);
    wAdiff          = wA - Accel2(3); FxwA = wAdiff*rho*Vol(ii,:)*CaRot(3);
    % Forces from fluid acceleration inertia
    FxuAf           = uA*Vol(ii,:)*rho;
    FxvAf           = vA*Vol(ii,:)*rho;
    FxwAf           = wA*Vol(ii,:)*rho;
    % Combine the forces and moments
    if ShiftCg(3) > 0
        F           = [0, 0, 0];
        M           = [0, 0, 0];
        FMt(ii,:)   = [F,M];
    else
        F           = [FxuV + FxuA + FxuAf,...
            FxvV + FxvA + FxvAf,...
            FxwV + FxwA + FxwAf];
        M           = cross(rRot,F);
        FMt(ii,:)   = [F,M];
    end
end
f  = [sum(FMt(:,1));sum(FMt(:,2));sum(FMt(:,3));sum(FMt(:,4));sum(FMt(:,5));sum(FMt(:,6))];

== matlab function Moorings/MooringMatrix/Structure/Motion Sensor/Angle ==
  data: Q input double; E output double
function E  = EulerAngle(Q)
%#codegen
E=zeros(3,1);
E(1) = atan2( (2*(Q(1)*Q(2)+Q(3)*Q(4))), (1-2* (Q(2)^2+Q(3)^2) ) );
E(2) = asin( 2* (Q(1)*Q(3) - Q(4)*Q(2)));
E(3) = atan2( (2*(Q(1)*Q(4)+Q(2)*Q(3))), (1-2* (Q(3)^2+Q(4)^2) ) );
